simulink model "Problem7"  (R2020b)
settings: Solver=FixedStepAuto  StartTime=0.0  StopTime=10.0  FixedStep=0.001  RelTol=1e-3
settings Model: Creator=ARPITA  LastModifiedBy=ARPITA

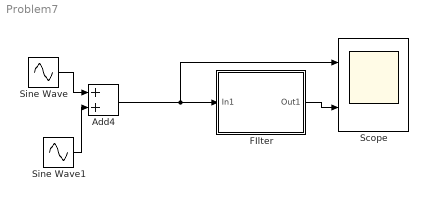
== system Problem7 ==
  Add4 : Sum
  FIlter : Subsystem  TreatAsAtomicUnit=on
  Scope : Scope  NumInputPorts=2
  Sine Wave : Sin  SampleTime=0
  Sine Wave1 : Sin  Amplitude=0.05  Frequency=200  SampleTime=0
  wires:
  Sine Wave1/1 -> Add4/2
  Sine Wave/1 -> Add4/1
  FIlter/1(Out1) -> Scope/2
  Add4/1 -> Scope/1, FIlter/1(In1)

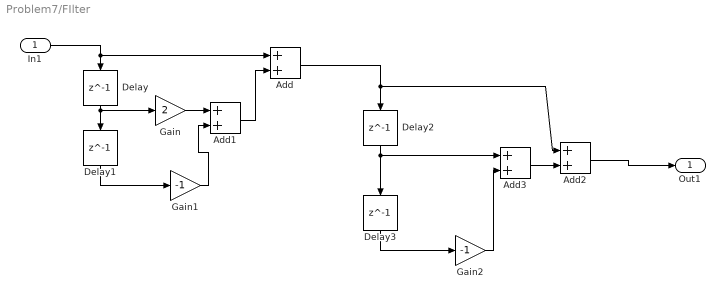
== system Problem7/FIlter ==
  In1 : Inport
  Add{,1..3} (4 alike) : Sum
  Delay{,1..3} (4 alike) : Delay  DelayLength=1
  Gain : Gain  Gain=2
  Gain1 : Gain  Gain=-1
  Gain2 : Gain  Gain=-1
  Out1 : Outport
  wires:
  Add3/1 -> Add2/2
  Delay2/1 -> Delay3/1, Add3/1
  Gain/1 -> Add1/1
  Delay/1 -> Delay1/1, Gain/1
  Gain2/1 -> Add3/2
  Gain1/1 -> Add1/2
  Delay1/1 -> Gain1/1
  Delay3/1 -> Gain2/1
  Add/1 -> Add2/1, Delay2/1
  Add1/1 -> Add/2
  In1/1 -> Delay/1, Add/1
  Add2/1 -> Out1/1
